simulink model "SEWSYS_Duplicate"  (Simulink 6.0)
settings: Solver=FixedStepDiscrete  SolverMode=SingleTasking  StartTime=0  StopTime=Q  FixedStep=1  RelTol=1e-3
PreLoadFcn:
  | helpdlg('After the simulation: run the file loadresults.m to load output data into MATLABs workspace. NOTE! All previous simulation data in subfolder Results is overwritten!')
values from neighbouring files (symbols this model uses):
  andpt = 1/3    (= 0.333333333333)    [constants.m]    (also in roadwear.m)
  andt = 0.15    [constants.m]    (also in roadwear.m = 0.1)
  baseflow = str2num(get(HH, 'String'))    [cal_inputs.m]
  BDT = [ ... (first row only)    [pollutants.m]
  BODofVS = 0.4    [sewageplant.m]
  delayinit = [zeros(1,nr_ex_H2O)]    [constants.m]
  Drainage = [ ... (first row only)    [pollutants.m]
  Faeces = [ ... (first row only)    [pollutants.m]
  fast = 0.7    [constants.m]    (also in roadwear.m = 0.5)
  Industry = [ ... (first row only)    [pollutants.m]
  K = a.*R.^b    [buildupwashoff.m]
  nr_ex_H2O = totnr-1    (= 20)    [cal_Prep.m]
  numberOfPersons = in_numberOfPersons    [cal_Prep.m]
  othermax = drydepmax*othera    [constants.m]
  ProcSS_bio = 0.01    [sewageplant.m]
  ProcSS_chem = 0.007    [sewageplant.m]
  ProcSS_presed = 0.025    [sewageplant.m]
  ProcSS_sand = 0.42*0.70    (= 0.294)    [sewageplant.m]
  ProcSS_screen = 0.185*0.85    (= 0.15725)    [sewageplant.m]
  roadaccmax = dryper*24*sph*fast*(p_tyrewear+p_roadwear+p_exhaust+p_breakwear+p_drydep+p_corrZn+p_oildischarge+p_catalyst)    [constants.m]
  roadkm = 63e9    (= 63000000000)    [constants.m]    (also in roadwear.m = 67000000000)
  roadrunpart = 1    [constants.m]
  roadwear = 130000    [constants.m]
  roofmax = (Znroofmax*RoofZna+Curoofmax*RoofCua)*roofrunpart+drydepmax*roofa    [constants.m]
  roofrunpart = 0.5    [constants.m]
  sec_per_ts = in_sec_per_ts    [cal_Prep.m]    (also in make_monthly_93_03.m = 600)
  spBiooxidBod = 0.5    [sewageplant.m]
  spBiored = 0.95    [sewageplant.m]
  spCcontent = 0.5424    [sewageplant.m]
  spChemFe = 0.171    [sewageplant.m]
  spChemicalPart = [ ... (first row only)    [sewageplant.m]
  spCODBOD = 2.51    [sewageplant.m]
  spDenSS = 0.25    [sewageplant.m]
  sph = 3600/sec_per_ts    [cal_Prep.m]
  spHeavym = [0.41 0.525 0.5 ... (first row only)    [sewageplant.m]
  spHjust = 1    [sewageplant.m]
  spN2ONpurEmitted = 0.0003    [sewageplant.m]
  spNemitted = 0.5    [sewageplant.m]
  spNitrif = 1.07    [sewageplant.m]
  spNpur = 1    [sewageplant.m]
  spOcontent = 0.3575    [sewageplant.m]
  spPBound = 0.97*0.5    (= 0.485)    [sewageplant.m]
  spPout = 0.38    [sewageplant.m]
  spPout1 = 0    [sewageplant.m]
  spVSofSS = 0.7    [sewageplant.m]
  SSred_bio = 0.65    [sewageplant.m]
  SSred_chem = 0.4    [sewageplant.m]
  SSred_presed = 0.75    [sewageplant.m]
  SSred_sand = 0.0032    [sewageplant.m]
  SSred_screen = 0.017    [sewageplant.m]
  SStoWater = 1E6    (= 1000000)    [sewageplant.m]
  totnr = 21    [cal_Prep.m]
  tyrewear = 9000    [constants.m]
  Urine = [ ... (first row only)    [pollutants.m]
  VSofSS_sand = 0.26    [sewageplant.m]
  VSofSS_screen = 0.60    (= 0.6)    [sewageplant.m]
  yearly_rain = in_yearly_rain    [cal_Prep.m]    (also in raininfo.m)
undefined symbols (not defined in the file or in its folder): brakep, catalystp, Curoofp, DiscIntNeverNeededParam, drydep, exhp, fkmday, init_init, init_time, nhv, oilp, othera, redu, roada, roadp, roadZna, roofa, RoofCua, RoofZna, sani, stormw, tota, tyrep, wetdep, Znroofp
libraries: simulink x2, SEWSYS_library x2
(part 2 of 2)

== system SEWSYS_Duplicate/Sewage plant/Sandpit/Separation/3-6 ==
  in_1 : Inport  Orientation=down  Port=1  LatchInput=off
  "in_2 " : Inport  Orientation=down  Port=2  LatchInput=off
  Ground2 : Ground  Orientation=down
  Mux : Mux  Orientation=down
  N-tot : MATLABFcn  Orientation=down  MATLABFcn=(u(1)-u(2)-u(3))*SSred_sand  OutputDimensions=1
  NH4 : Product  Orientation=down  SaturateOnIntegerOverflow=on  InputSameDT=on
  "NH4 " : Fcn  Orientation=down  Expr=u(2)
  NH5 : Product  Orientation=down  SaturateOnIntegerOverflow=on  InputSameDT=on
  NO3 : Fcn  Orientation=down  Expr=u(3)
  Sum : Sum  Orientation=down  Inputs=+++  SaturateOnIntegerOverflow=on  InputSameDT=on
  out_1 : Outport  Orientation=down  InitialOutput=0
  wires:
  Ground2/1 -> Mux/4
  NH5/1 -> Mux/3, Sum/3
  "in_2 "/1 -> N-tot/1, "NH4 "/1, NO3/1
  NO3/1 -> NH5/2
  "NH4 "/1 -> NH4/2
  Sum/1 -> Mux/1
  N-tot/1 -> Sum/1
  Mux/1 -> out_1/1
  in_1/1 -> NH4/1, NH5/1
  NH4/1 -> Sum/2, Mux/2

== system SEWSYS_Duplicate/Sewage plant/Sandpit/Separation/if u>0 then 1/u else 0 ==
  note: if u<=0, 0, else 1/u, end
  in_1 : Inport  Orientation=left  Port=1  LatchInput=off
  Constant : Constant  Orientation=left  Value=0
  Constant1 : Constant  Orientation=left
  Switch : Switch  Orientation=left  SaturateOnIntegerOverflow=on  InputSameDT=on
  Switch1 : Switch  Orientation=left  SaturateOnIntegerOverflow=on  InputSameDT=on
  inv. : Fcn  Orientation=left  Expr=1/u
  neg : Gain  Orientation=left  Gain=-1  SaturateOnIntegerOverflow=on
  neg1 : Gain  Orientation=left  Gain=-1  SaturateOnIntegerOverflow=on
  out_1 : Outport  Orientation=left  InitialOutput=0
  wires:
  Switch/1 -> out_1/1
  neg/1 -> Switch/2
  Constant/1 -> Switch/1
  inv./1 -> Switch/3
  Switch1/1 -> inv./1
  neg1/1 -> Switch1/2
  Constant1/1 -> Switch1/1
  in_1/1 -> neg/1, neg1/1, Switch1/3

== system SEWSYS_Duplicate/Sewage plant/Screen/Separation/3-6 ==
  in_1 : Inport  Orientation=down  Port=1  LatchInput=off
  "in_2 " : Inport  Orientation=down  Port=2  LatchInput=off
  Ground : Ground  Orientation=down
  Mux : Mux  Orientation=down
  N-tot : MATLABFcn  Orientation=down  MATLABFcn=(u(1)-u(2)-u(3))*SSred_screen  OutputDimensions=1
  NH4 : Product  Orientation=down  SaturateOnIntegerOverflow=on  InputSameDT=on
  "NH4 " : Fcn  Orientation=down  Expr=u(2)
  NH5 : Product  Orientation=down  SaturateOnIntegerOverflow=on  InputSameDT=on
  NO3 : Fcn  Orientation=down  Expr=u(3)
  Sum : Sum  Orientation=down  Inputs=+++  SaturateOnIntegerOverflow=on  InputSameDT=on
  out_1 : Outport  Orientation=down  InitialOutput=0
  wires:
  NH4/1 -> Mux/2, Sum/2
  in_1/1 -> NH5/1, NH4/1
  Mux/1 -> out_1/1
  N-tot/1 -> Sum/1
  Sum/1 -> Mux/1
  "NH4 "/1 -> NH4/2
  NO3/1 -> NH5/2
  "in_2 "/1 -> NO3/1, "NH4 "/1, N-tot/1
  NH5/1 -> Sum/3, Mux/3
  Ground/1 -> Mux/4

== system SEWSYS_Duplicate/Sewage plant/Screen/Separation/if u>0 then 1/u else 0 ==
  note: if u<=0, 0, else 1/u, end
  in_1 : Inport  Orientation=left  Port=1  LatchInput=off
  Constant : Constant  Orientation=left  Value=0
  Constant1 : Constant  Orientation=left
  Switch : Switch  Orientation=left  SaturateOnIntegerOverflow=on  InputSameDT=on
  Switch1 : Switch  Orientation=left  SaturateOnIntegerOverflow=on  InputSameDT=on
  inv. : Fcn  Orientation=left  Expr=1/u
  neg : Gain  Orientation=left  Gain=-1  SaturateOnIntegerOverflow=on
  neg1 : Gain  Orientation=left  Gain=-1  SaturateOnIntegerOverflow=on
  out_1 : Outport  Orientation=left  InitialOutput=0
  wires:
  Constant/1 -> Switch/1
  neg/1 -> Switch/2
  Switch/1 -> out_1/1
  inv./1 -> Switch/3
  Switch1/1 -> inv./1
  neg1/1 -> Switch1/2
  Constant1/1 -> Switch1/1
  in_1/1 -> neg/1, neg1/1, Switch1/3

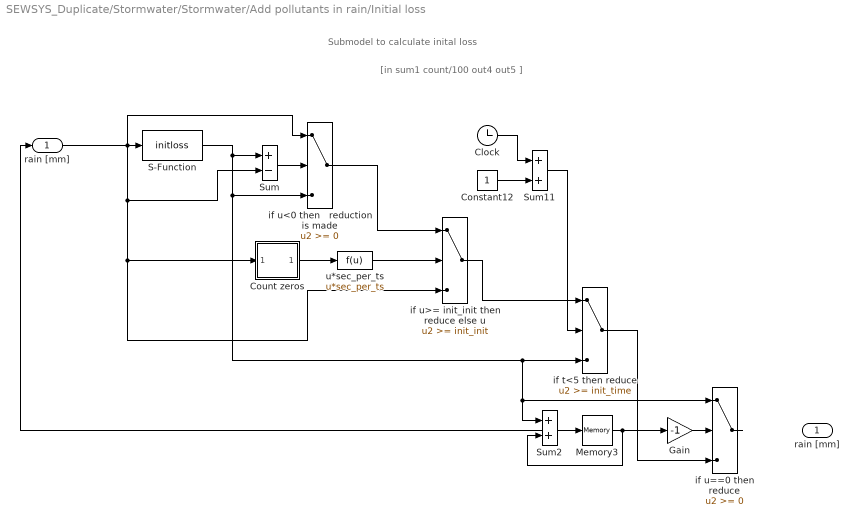
== system SEWSYS_Duplicate/Stormwater/Stormwater/Add pollutants in rain/Initial loss ==
  note: Submodel to calculate inital loss
  note: [in sum1 count/100 out4 out5 ]
  rain [mm] : Inport  Port=1  LatchInput=off
  Clock : Clock
      settings: Decimation=10
  Constant12 : Constant
  Count zeros : Subsystem
  Gain : Gain  Gain=-1  SaturateOnIntegerOverflow=on
  Memory3 : Memory
  S-Function : S-Function  FunctionName=initloss  Parameters=init
  Sum : Sum  Inputs=+-  SaturateOnIntegerOverflow=on  InputSameDT=on
  Sum11 : Sum  SaturateOnIntegerOverflow=on  InputSameDT=on
  Sum2 : Sum  SaturateOnIntegerOverflow=on  InputSameDT=on
  if t<5 then reduce : Switch  Threshold=init_time  SaturateOnIntegerOverflow=on  InputSameDT=on
  if u<0 then   reduction is made : Switch  SaturateOnIntegerOverflow=on  InputSameDT=on
  if u==0 then reduce : Switch  SaturateOnIntegerOverflow=on  InputSameDT=on
  if u>= init_init then reduce else u : Switch  Threshold=init_init  SaturateOnIntegerOverflow=on  InputSameDT=on
  u*sec_per_ts : Fcn  Expr=u*sec_per_ts
  rain [mm] : Outport
  wires:
  S-Function/1 -> Sum/1, if u<0 then   reduction is made/3, if t<5 then reduce/3, if u==0 then reduce/1, Sum2/1
  Sum11/1 -> if t<5 then reduce/2
  Sum/1 -> if u<0 then   reduction is made/2
  if u<0 then   reduction is made/1 -> if u>= init_init then reduce else u/1
  rain [mm]/1 -> Count zeros/1(In1), if u>= init_init then reduce else u/3, Sum/2, S-Function/1, if u<0 then   reduction is made/1
  Count zeros/1(Out1) -> u*sec_per_ts/1
  u*sec_per_ts/1 -> if u>= init_init then reduce else u/2
  Clock/1 -> Sum11/1
  Constant12/1 -> Sum11/2
  Gain/1 -> if u==0 then reduce/2
  if u==0 then reduce/1 -> rain [mm]/1
  Memory3/1 -> Gain/1, Sum2/2
  Sum2/1 -> Memory3/1
  if u>= init_init then reduce else u/1 -> if t<5 then reduce/1
  if t<5 then reduce/1 -> if u==0 then reduce/3

== system SEWSYS_Duplicate/Stormwater/Stormwater/Add pollutants in rain/wet deposition ==
  rain [mm] : Inport  Port=1  LatchInput=off
  Mux : Mux  Inputs=2
  Product1 : Product  SaturateOnIntegerOverflow=on  InputSameDT=on
  Product2 : Product  Inputs=*/  SaturateOnIntegerOverflow=on  InputSameDT=on
  To File : ToFile  Filename=Results\s_wetdep.mat  MatrixName=s_wetdep
      settings: Decimation=store1_yes
  To Workspace6 : ToWorkspace  VariableName=s_wetdep  SampleTime=-1  SaveFormat=Array
      settings: MaxDataPoints=lim_off
  rain mm/yr : Constant  Value=yearly_rain
  wet deposition ug/m2*yr : Constant  Value=wetdep
  rain [mm] pollutants [ug/m2] : Outport
  wires:
  rain [mm]/1 -> Product1/1, Mux/1
  Product2/1 -> Product1/2
  wet deposition ug/m2*yr/1 -> Product2/1
  rain mm/yr/1 -> Product2/2
  Product1/1 -> Mux/2
  Mux/1 -> rain [mm] pollutants [ug/m2]/1, To Workspace6/1, To File/1

== system SEWSYS_Duplicate/Stormwater/Stormwater/Rain -> Stormwater/other surfaces ==
  rain[mm] pollutants [ug/m2] : Inport  Port=1  LatchInput=off
  Demux2 : Demux  Outputs=[1 -1]
  Mux2 : Mux  Inputs=2
  Product1 : Product  SaturateOnIntegerOverflow=on  InputSameDT=on
  Sum : Sum  Inputs=|++  SaturateOnIntegerOverflow=on  InputSameDT=on
  To File : ToFile  Filename=Results\s_other.mat  MatrixName=s_other
      settings: Decimation=store1_yes
  To Workspace7 : ToWorkspace  VariableName=s_other  SampleTime=-1  SaveFormat=Array
      settings: MaxDataPoints=lim_off
  ackumulation and wash-off : Subsystem
  area [m2] : Constant  Value=othera
  dry deposition : Subsystem
  rain on other surfaces : Subsystem
  ug - g : Gain  Gain=0.000001  SaturateOnIntegerOverflow=on
  rain[m3] pollutants [g] : Outport
  wires:
  rain[mm] pollutants [ug/m2]/1 -> Demux2/1
  Mux2/1 -> rain[m3] pollutants [g]/1
  area [m2]/1 -> Product1/2
  Demux2/2 -> Product1/1
  Demux2/1 -> ackumulation and wash-off/1(rain [mm]), rain on other surfaces/1(rain [mm])
  dry deposition/1(pollutants [ug]) -> ackumulation and wash-off/2(pollutant [ug])
  Product1/1 -> Sum/2
  rain on other surfaces/1(rain [m3]) -> Mux2/1
  Sum/1 -> ug - g/1
  ug - g/1 -> Mux2/2
  ackumulation and wash-off/1(pollutants [ug]) -> Sum/1, To Workspace7/1, To File/1

== system SEWSYS_Duplicate/Stormwater/Stormwater/Rain -> Stormwater/road surfaces ==
  rain [mm] pollutants [ug/m2] : Inport  Port=1  LatchInput=off
  Demux1 : Demux  Outputs=[1 -1]
  Mux3 : Mux  Inputs=2
  Sum1 : Sum  Inputs=|++  SaturateOnIntegerOverflow=on  InputSameDT=on
  To File : ToFile  Filename=Results\s_road.mat  MatrixName=s_road
      settings: Decimation=store1_yes
  To Workspace7 : ToWorkspace  VariableName=s_road  SampleTime=-1  SaveFormat=Array
      settings: MaxDataPoints=lim_off
  To Workspace8 : ToWorkspace  VariableName=roadpoll  SampleTime=-1  SaveFormat=Array
      settings: MaxDataPoints=lim_off
  accumulation and wash-off : Subsystem
  pollutants on roads : Subsystem
  rain on road : Subsystem
  ug - g : Gain  Gain=0.000001  SaturateOnIntegerOverflow=on
  rain[m3] pollutants [g] : Outport
  wires:
  rain on road/1(rain [m3]) -> Mux3/1
  accumulation and wash-off/1(rain [mm]1) -> rain on road/1(rain [mm])
  Demux1/2 -> rain on road/2(pollutants [ug/m2])
  Demux1/1 -> accumulation and wash-off/1(rain [mm])
  rain [mm] pollutants [ug/m2]/1 -> Demux1/1
  Mux3/1 -> rain[m3] pollutants [g]/1
  rain on road/2(pollutants [ug]) -> Sum1/1
  accumulation and wash-off/2(pollutants [ug]) -> Sum1/2, To Workspace7/1, To File/1
  Sum1/1 -> ug - g/1
  ug - g/1 -> Mux3/2
  pollutants on roads/1(pollutants[ ug]) -> accumulation and wash-off/2(pollutant [ug]), To Workspace8/1

== system SEWSYS_Duplicate/Stormwater/Stormwater/Rain -> Stormwater/roofs ==
  note: Accumulates pollutants over time. Washes out during rain.
  rain [mm]  pollutants[ug/m2] : Inport  Port=1  LatchInput=off
  Demux : Demux  Outputs=[1 -1]
  Mux : Mux  Inputs=2
  Pollutants on roofs : Subsystem
  Product : Product  SaturateOnIntegerOverflow=on  InputSameDT=on
  Sum : Sum  Inputs=|++  SaturateOnIntegerOverflow=on  InputSameDT=on
  To File : ToFile  Filename=Results\s_roof.mat  MatrixName=s_roof
      settings: Decimation=store1_yes
  To Workspace7 : ToWorkspace  VariableName=s_roof  SampleTime=-1  SaveFormat=Array
      settings: MaxDataPoints=lim_off
  ackumulation and wash-off : Subsystem
  area [m2] : Constant  Value=roofa
  rain on roof surfaces : Subsystem
  ug - g : Gain  Gain=0.000001  SaturateOnIntegerOverflow=on
  rain[m3] pollutants [g] : Outport
  wires:
  Mux/1 -> rain[m3] pollutants [g]/1
  area [m2]/1 -> Product/2
  Demux/2 -> Product/1
  rain on roof surfaces/1(rain [m3]) -> Mux/1
  rain [mm]  pollutants[ug/m2]/1 -> Demux/1
  Product/1 -> Sum/2
  Sum/1 -> ug - g/1
  ug - g/1 -> Mux/2
  Demux/1 -> rain on roof surfaces/1(rain [mm]), ackumulation and wash-off/1(rain [mm])
  ackumulation and wash-off/1(pollutants [ug]) -> Sum/1, To Workspace7/1, To File/1
  Pollutants on roofs/1(pollutants [ug]) -> ackumulation and wash-off/2(pollutant [ug])

== system SEWSYS_Duplicate/Stormwater/Stormwater/Runoff/Make per second ==
  In1 : Inport  Port=1  LatchInput=off
  Demux : Demux  Outputs=[1 -1]
  Mux1 : Mux  Inputs=2
  g - g/s : Gain  Gain=1/sec_per_ts  SaturateOnIntegerOverflow=on
  m3 - m3/s : Gain  Gain=1/sec_per_ts  SaturateOnIntegerOverflow=on
  Out1 : Outport
  wires:
  In1/1 -> Demux/1
  Mux1/1 -> Out1/1
  Demux/1 -> m3 - m3/s/1
  m3 - m3/s/1 -> Mux1/1
  Demux/2 -> g - g/s/1
  g - g/s/1 -> Mux1/2

== system SEWSYS_Duplicate/Stormwater/Stormwater/Runoff/Subsystem1 ==
  In1 : Inport  Port=1  LatchInput=off
  Gain : Gain  Gain=sec_per_ts  SaturateOnIntegerOverflow=on
  Qut : Fcn  Expr=tota*K*u^(5/3)
  Sum : Sum  SaturateOnIntegerOverflow=on  InputSameDT=on
  Sum1 : Sum  Inputs=+-  SaturateOnIntegerOverflow=on  InputSameDT=on
  Sum2 : Sum  SaturateOnIntegerOverflow=on  InputSameDT=on
  Unit Delay1 : UnitDelay  Orientation=left
  Unit Delay2 : UnitDelay
  if u>0 then u else 1 : Subsystem
      mask Display: disp('1/u')
  y : Fcn  Expr=u/tota
  yprim : Fcn  Expr=u*sec_per_ts/tota/3
  Out1 : Outport
  wires:
  Qut/1 -> Sum1/2, Out1/1
  Unit Delay1/1 -> Sum2/2
  Sum2/1 -> Unit Delay1/1, y/1
  Gain/1 -> Sum2/1
  Sum1/1 -> Gain/1
  y/1 -> if u>0 then u else 1/1(in_1)
  yprim/1 -> Sum/1
  Sum/1 -> Qut/1
  if u>0 then u else 1/1(out_1) -> Unit Delay2/1
  Unit Delay2/1 -> Sum/2
  In1/1 -> Sum1/1, yprim/1

== system SEWSYS_Duplicate/Sewage plant/Biological stage/Predenitri- fication/N-org to NH4 through oxid to CO2/if u>0 then 1/u else 0 ==
  note: if u<=0, 0, else 1/u, end
  in_1 : Inport  Orientation=left  Port=1  LatchInput=off
  Constant : Constant  Orientation=left  Value=0
  Constant1 : Constant  Orientation=left
  Switch : Switch  Orientation=left  SaturateOnIntegerOverflow=on  InputSameDT=on
  Switch1 : Switch  Orientation=left  SaturateOnIntegerOverflow=on  InputSameDT=on
  inv. : Fcn  Orientation=left  Expr=1/u
  neg : Gain  Orientation=left  Gain=-1  SaturateOnIntegerOverflow=on
  out_1 : Outport  Orientation=left  InitialOutput=0
  wires:
  Constant1/1 -> Switch1/1
  in_1/1 -> Switch1/3, neg/1
  neg/1 -> Switch1/2, Switch/2
  Switch1/1 -> inv./1
  Switch/1 -> out_1/1
  inv./1 -> Switch/3
  Constant/1 -> Switch/1

== system SEWSYS_Duplicate/Sewage plant/Biological stage/Predenitri- fication/NH3 emissions from  aeration to nitrification  and degration of BOD./if u>0 then 1/u else 0 ==
  note: if u<=0, 0, else 1/u, end
  in_1 : Inport  Orientation=left  Port=1  LatchInput=off
  Constant : Constant  Orientation=left  Value=0
  Constant1 : Constant  Orientation=left
  Switch : Switch  Orientation=left  SaturateOnIntegerOverflow=on  InputSameDT=on
  Switch1 : Switch  Orientation=left  SaturateOnIntegerOverflow=on  InputSameDT=on
  inv. : Fcn  Orientation=left  Expr=1/u
  neg : Gain  Orientation=left  Gain=-1  SaturateOnIntegerOverflow=on
  out_1 : Outport  Orientation=left  InitialOutput=0
  wires:
  Constant1/1 -> Switch1/1
  in_1/1 -> Switch1/3, neg/1
  neg/1 -> Switch1/2, Switch/2
  Switch1/1 -> inv./1
  Switch/1 -> out_1/1
  inv./1 -> Switch/3
  Constant/1 -> Switch/1

== system SEWSYS_Duplicate/Sewage plant/Biological stage/Predenitri- fication/NH3 emissions from  aeration to nitrification  and degration of BOD./if u>0 then 1/u else 1 ==
  note: if u<=0, 0, else 1/u, end
  in_1 : Inport  Orientation=left  Port=1  LatchInput=off
  Constant : Constant  Orientation=left  Value=0
  Constant1 : Constant  Orientation=left
  Switch : Switch  Orientation=left  SaturateOnIntegerOverflow=on  InputSameDT=on
  Switch1 : Switch  Orientation=left  SaturateOnIntegerOverflow=on  InputSameDT=on
  inv. : Fcn  Orientation=left  Expr=1/u
  neg : Gain  Orientation=left  Gain=-1  SaturateOnIntegerOverflow=on
  out_1 : Outport  Orientation=left  InitialOutput=0
  wires:
  Constant1/1 -> Switch1/1
  in_1/1 -> Switch1/3, neg/1
  neg/1 -> Switch1/2, Switch/2
  Switch1/1 -> inv./1
  Switch/1 -> out_1/1
  inv./1 -> Switch/3
  Constant/1 -> Switch/1

== system SEWSYS_Duplicate/Sewage plant/Biological stage/Predenitri- fication/Nitrification/ denitrification/N-org to NH4 ==
  In1 : Inport  Orientation=down  Port=1  LatchInput=off
  In2 : Inport  Orientation=down  Port=2  LatchInput=off
  C-tot : Fcn  Orientation=down  Expr=u(10)
  Ctot degr. : Fcn  Orientation=down  Expr=u(10)
  N-org : Fcn  Orientation=down  Expr=u(3)-u(4)-u(5)
  N-org degraded  to NH4 : Product  Orientation=down  SaturateOnIntegerOverflow=on  InputSameDT=on
  NH4 increased : MATLABFcn  Orientation=down  MATLABFcn=[zeros(3,1); u ; zeros(17,1)]  OutputDimensions=totnr
  Part of C-tot degraded : Product  Orientation=down  SaturateOnIntegerOverflow=on  InputSameDT=on
  if u>0 then 1/u else 0 : Subsystem  Orientation=down
      mask Display: disp('1/u')
  Out1 : Outport  Orientation=down  InitialOutput=0
  wires:
  Ctot degr./1 -> Part of C-tot degraded/1
  In1/1 -> Ctot degr./1
  C-tot/1 -> if u>0 then 1/u else 0/1(in_1)
  if u>0 then 1/u else 0/1(out_1) -> Part of C-tot degraded/2
  In2/1 -> C-tot/1, N-org/1
  N-org/1 -> N-org degraded  to NH4/2
  N-org degraded  to NH4/1 -> NH4 increased/1
  NH4 increased/1 -> Out1/1
  Part of C-tot degraded/1 -> N-org degraded  to NH4/1

== system SEWSYS_Duplicate/Stormwater/Stormwater/Add pollutants in rain/Initial loss/Count zeros ==
  In1 : Inport  Port=1  LatchInput=off
  Constant13 : Constant  Value=0
  Constant8 : Constant
  Counter1 : Subsystem  TreatAsAtomicUnit=on
  Gain1 : Gain  Gain=-1  SaturateOnIntegerOverflow=on
  Memory1 : Memory
  if u== 0 then 1 else 1 : Switch  SaturateOnIntegerOverflow=on  InputSameDT=on
  Out1 : Outport
  wires:
  if u== 0 then 1 else 1/1 -> Counter1/Enable
  Counter1/1(Out1) -> Memory1/1
  Constant8/1 -> if u== 0 then 1 else 1/1
  Gain1/1 -> if u== 0 then 1 else 1/2
  Constant13/1 -> if u== 0 then 1 else 1/3
  In1/1 -> Gain1/1
  Memory1/1 -> Out1/1

== system SEWSYS_Duplicate/Stormwater/Stormwater/Rain -> Stormwater/other surfaces/ackumulation and wash-off ==
  rain [mm] : Inport  Port=1  LatchInput=off
  pollutant [ug] : Inport  Port=2  LatchInput=off
  Demux1 : Demux  Outputs=[1 -1]
  Mux : Mux  Inputs=2
  Mux1 : Mux  Inputs=3
  Specify initial condition here : UnitDelay  Orientation=left  X0=othermax
  Terminator : Terminator
  Unit Delay : UnitDelay  Orientation=left  X0=delayinit
  ackumulation Fcn1 : MATLABFcn  MATLABFcn=ackumulation  OutputDimensions=nr_ex_H2O
  deltaP : Scope
      settings: YMin=0  YMax=2250
  washoff Fcn : MATLABFcn  MATLABFcn=washoff  OutputDimensions=totnr
  pollutants [ug] : Outport
  wires:
  washoff Fcn/1 -> Demux1/1
  Demux1/2 -> deltaP/1, Unit Delay/1, pollutants [ug]/1
  Mux/1 -> washoff Fcn/1
  Unit Delay/1 -> Mux1/2
  Specify initial condition here/1 -> Mux1/3
  ackumulation Fcn1/1 -> Mux/2, Specify initial condition here/1
  Demux1/1 -> Terminator/1
  rain [mm]/1 -> Mux/1
  Mux1/1 -> ackumulation Fcn1/1
  pollutant [ug]/1 -> Mux1/1

== system SEWSYS_Duplicate/Stormwater/Stormwater/Rain -> Stormwater/other surfaces/dry deposition ==
  Product : Product  Inputs=*/  SaturateOnIntegerOverflow=on  InputSameDT=on
  Product1 : Product  SaturateOnIntegerOverflow=on  InputSameDT=on
  area m2 : Constant  Orientation=up  Value=othera
  timesteps/yr : Constant  Value=365*24*sph
  torrdep ug/m2*yr : Constant  Value=drydep
  pollutants [ug] : Outport
  wires:
  area m2/1 -> Product1/2
  Product1/1 -> pollutants [ug]/1
  Product/1 -> Product1/1
  torrdep ug/m2*yr/1 -> Product/1
  timesteps/yr/1 -> Product/2

== system SEWSYS_Duplicate/Stormwater/Stormwater/Rain -> Stormwater/other surfaces/rain on other surfaces ==
  rain [mm] : Inport  Port=1  LatchInput=off
  Product1 : Product  SaturateOnIntegerOverflow=on  InputSameDT=on
  area [m2] : Constant  Value=othera
  mm->m : Gain  Gain=0.001  SaturateOnIntegerOverflow=on
  rain [m3] : Outport
  wires:
  mm->m/1 -> Product1/1
  rain [mm]/1 -> mm->m/1
  area [m2]/1 -> Product1/2
  Product1/1 -> rain [m3]/1

== system SEWSYS_Duplicate/Stormwater/Stormwater/Rain -> Stormwater/road surfaces/accumulation and wash-off ==
  rain [mm] : Inport  Port=1  LatchInput=off
  pollutant [ug] : Inport  Port=2  LatchInput=off
  Demux1 : Demux  Outputs=[1 -1]
  Mux : Mux  Inputs=2
  Mux1 : Mux  Inputs=3
  Specify initial condition here : UnitDelay  Orientation=left  X0=roadaccmax
  To Workspace7 : ToWorkspace  VariableName=acc  SampleTime=-1  SaveFormat=Array
      settings: MaxDataPoints=lim_off
  Unit Delay : UnitDelay  Orientation=left  X0=delayinit
  ackumulation Fcn1 : MATLABFcn  MATLABFcn=ackumulation  OutputDimensions=nr_ex_H2O
  washoff Fcn : MATLABFcn  MATLABFcn=washoff  OutputDimensions=totnr
  rain [mm]1 : Outport
  pollutants [ug] : Outport  Port=2
  wires:
  Demux1/1 -> rain [mm]1/1
  pollutant [ug]/1 -> Mux1/1
  ackumulation Fcn1/1 -> Specify initial condition here/1, Mux/2, To Workspace7/1
  Specify initial condition here/1 -> Mux1/3
  Mux1/1 -> ackumulation Fcn1/1
  Unit Delay/1 -> Mux1/2
  Mux/1 -> washoff Fcn/1
  washoff Fcn/1 -> Demux1/1
  rain [mm]/1 -> Mux/1
  Demux1/2 -> Unit Delay/1, pollutants [ug]/1

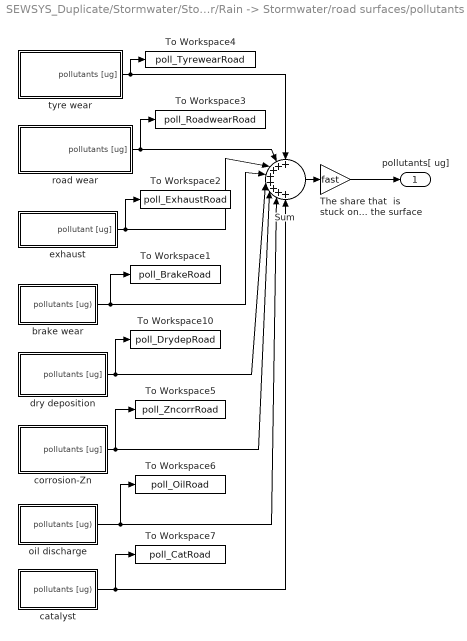
== system SEWSYS_Duplicate/Stormwater/Stormwater/Rain -> Stormwater/road surfaces/pollutants on roads ==
  Sum : Sum  Inputs=++++++++  SaturateOnIntegerOverflow=on  InputSameDT=on
  The share that  is stuck on the surface : Gain  Gain=fast  SaturateOnIntegerOverflow=on
  To Workspace1 : ToWorkspace  VariableName=poll_BrakeRoad  SampleTime=-1  SaveFormat=Array
      settings: MaxDataPoints=10
  To Workspace10 : ToWorkspace  VariableName=poll_DrydepRoad  SampleTime=-1  SaveFormat=Array
      settings: MaxDataPoints=10
  To Workspace2 : ToWorkspace  VariableName=poll_ExhaustRoad  SampleTime=-1  SaveFormat=Array
      settings: MaxDataPoints=10
  To Workspace3 : ToWorkspace  VariableName=poll_RoadwearRoad  SampleTime=-1  SaveFormat=Array
      settings: MaxDataPoints=10
  To Workspace4 : ToWorkspace  VariableName=poll_TyrewearRoad  SampleTime=-1  SaveFormat=Array
      settings: MaxDataPoints=10
  To Workspace5 : ToWorkspace  VariableName=poll_ZncorrRoad  SampleTime=-1  SaveFormat=Array
      settings: MaxDataPoints=10
  To Workspace6 : ToWorkspace  VariableName=poll_OilRoad  SampleTime=-1  SaveFormat=Array
      settings: MaxDataPoints=10
  To Workspace7 : ToWorkspace  VariableName=poll_CatRoad  SampleTime=-1  SaveFormat=Array
      settings: MaxDataPoints=10
  brake wear : Subsystem
  catalyst : Subsystem
  corrosion-Zn : Subsystem
  dry deposition : Subsystem
  exhaust : Subsystem
  oil discharge : Subsystem
  road wear : Subsystem
  tyre wear : Subsystem
  pollutants[ ug] : Outport
  wires:
  Sum/1 -> The share that  is stuck on the surface/1
  The share that  is stuck on the surface/1 -> pollutants[ ug]/1
  tyre wear/1(pollutants [ug]) -> Sum/1, To Workspace4/1
  road wear/1(pollutants [ug]) -> Sum/2, To Workspace3/1
  exhaust/1(pollutant [ug]) -> Sum/3, To Workspace2/1
  brake wear/1("pollutants [ug) ") -> Sum/4, To Workspace1/1
  dry deposition/1(pollutants [ug]) -> Sum/5, To Workspace10/1
  corrosion-Zn/1(pollutants [ug]) -> Sum/6, To Workspace5/1
  oil discharge/1("pollutants [ug) ") -> Sum/7, To Workspace6/1
  catalyst/1("pollutants [ug) ") -> Sum/8, To Workspace7/1

== system SEWSYS_Duplicate/Stormwater/Stormwater/Rain -> Stormwater/road surfaces/rain on road ==
  note: [m]
  rain [mm] : Inport  Port=1  LatchInput=off
  pollutants [ug/m2] : Inport  Port=2  LatchInput=off
  Gain : Gain  Gain=0.001  SaturateOnIntegerOverflow=on
  Product : Product  SaturateOnIntegerOverflow=on  InputSameDT=on
  Product1 : Product  SaturateOnIntegerOverflow=on  InputSameDT=on
  area [m2] : Constant  Value=roada
  rain [m3] : Outport
  pollutants [ug] : Outport  Port=2
  wires:
  Product1/1 -> pollutants [ug]/1
  pollutants [ug/m2]/1 -> Product1/2
  area [m2]/1 -> Product1/1, Product/2
  rain [mm]/1 -> Gain/1
  Gain/1 -> Product/1
  Product/1 -> rain [m3]/1

== system SEWSYS_Duplicate/Stormwater/Stormwater/Rain -> Stormwater/roofs/Pollutants on roofs ==
  Corrosion-Cu : Subsystem
  Corrosion-Zn : Subsystem
  Sum : Sum  Inputs=+++  SaturateOnIntegerOverflow=on  InputSameDT=on
  To Workspace10 : ToWorkspace  VariableName=poll_DrydepRoof  SampleTime=-1  SaveFormat=Array
      settings: MaxDataPoints=10
  To Workspace11 : ToWorkspace  VariableName=poll_ZnRoof  SampleTime=-1  SaveFormat=Array
      settings: MaxDataPoints=10
  To Workspace9 : ToWorkspace  VariableName=poll_CuRoof  SampleTime=-1  SaveFormat=Array
      settings: MaxDataPoints=10
  dry deposition : Subsystem
  pollutants [ug] : Outport
  wires:
  Sum/1 -> pollutants [ug]/1
  Corrosion-Cu/1(pollutants [ug]) -> Sum/2, To Workspace9/1
  Corrosion-Zn/1(pollutants [ug]) -> Sum/3, To Workspace11/1
  dry deposition/1(pollutants [ug]) -> Sum/1, To Workspace10/1

== system SEWSYS_Duplicate/Stormwater/Stormwater/Rain -> Stormwater/roofs/ackumulation and wash-off ==
  rain [mm] : Inport  Port=1  LatchInput=off
  pollutant [ug] : Inport  Port=2  LatchInput=off
  Demux1 : Demux  Outputs=[1 -1]
  Mux : Mux  Inputs=2
  Mux1 : Mux  Inputs=3
  Specify initial condition here : UnitDelay  Orientation=left  X0=roofmax
  Terminator : Terminator
  Unit Delay : UnitDelay  Orientation=left  X0=delayinit
  ackumulation Fcn1 : MATLABFcn  MATLABFcn=ackumulation  OutputDimensions=nr_ex_H2O
  deltaP : Scope
      settings: TimeRange=50  YMin=0  YMax=1e+07
  washoff Fcn : MATLABFcn  MATLABFcn=washoff  OutputDimensions=totnr
  pollutants [ug] : Outport
  wires:
  Demux1/1 -> Terminator/1
  ackumulation Fcn1/1 -> Mux/2, Specify initial condition here/1
  Specify initial condition here/1 -> Mux1/3
  Unit Delay/1 -> Mux1/2
  Mux/1 -> washoff Fcn/1
  Demux1/2 -> pollutants [ug]/1, Unit Delay/1, deltaP/1
  washoff Fcn/1 -> Demux1/1
  Mux1/1 -> ackumulation Fcn1/1
  pollutant [ug]/1 -> Mux1/1
  rain [mm]/1 -> Mux/1

== system SEWSYS_Duplicate/Stormwater/Stormwater/Rain -> Stormwater/roofs/rain on roof surfaces ==
  rain [mm] : Inport  Port=1  LatchInput=off
  Product1 : Product  SaturateOnIntegerOverflow=on  InputSameDT=on
  area [m2] : Constant  Value=roofa
  mm->m : Gain  Gain=0.001  SaturateOnIntegerOverflow=on
  rain [m3] : Outport
  wires:
  Product1/1 -> rain [m3]/1
  area [m2]/1 -> Product1/2
  rain [mm]/1 -> mm->m/1
  mm->m/1 -> Product1/1

== system SEWSYS_Duplicate/Stormwater/Stormwater/Runoff/Subsystem1/if u>0 then u else 1 ==
  note: if u<=0, 0, else u, end
  in_1 : Inport  Port=1  LatchInput=off
  Constant : Constant  Value=0
  Switch : Switch  SaturateOnIntegerOverflow=on  InputSameDT=on
  inv. : Fcn  Expr=u
  neg : Gain  Gain=-1  SaturateOnIntegerOverflow=on
  out_1 : Outport  InitialOutput=0
  wires:
  Switch/1 -> out_1/1
  Constant/1 -> Switch/1
  neg/1 -> Switch/2
  inv./1 -> Switch/3
  in_1/1 -> neg/1, inv./1

== system SEWSYS_Duplicate/Sewage plant/Biological stage/Predenitri- fication/Nitrification/ denitrification/N-org to NH4/if u>0 then 1/u else 0 ==
  note: if u<=0, 0, else 1/u, end
  in_1 : Inport  Orientation=left  Port=1  LatchInput=off
  Constant : Constant  Orientation=left  Value=0
  Constant1 : Constant  Orientation=left
  Switch : Switch  Orientation=left  SaturateOnIntegerOverflow=on  InputSameDT=on
  Switch1 : Switch  Orientation=left  SaturateOnIntegerOverflow=on  InputSameDT=on
  inv. : Fcn  Orientation=left  Expr=1/u
  neg : Gain  Orientation=left  Gain=-1  SaturateOnIntegerOverflow=on
  out_1 : Outport  Orientation=left  InitialOutput=0
  wires:
  Constant1/1 -> Switch1/1
  in_1/1 -> Switch1/3, neg/1
  neg/1 -> Switch1/2, Switch/2
  Switch1/1 -> inv./1
  Switch/1 -> out_1/1
  inv./1 -> Switch/3
  Constant/1 -> Switch/1

== system SEWSYS_Duplicate/Stormwater/Stormwater/Add pollutants in rain/Initial loss/Count zeros/Counter1 ==
  Enable : EnablePort  StatesWhenEnabling=reset
  Constant7 : Constant
  Discrete-Time Integrator : DiscreteIntegrator  InitialCondition=1  ICPrevOutput=DiscIntNeverNeededParam  ICPrevScaledInput=DiscIntNeverNeededParam
  Out1 : Outport  InitialOutput=0
  wires:
  Discrete-Time Integrator/1 -> Out1/1
  Constant7/1 -> Discrete-Time Integrator/1

== system SEWSYS_Duplicate/Stormwater/Stormwater/Rain -> Stormwater/road surfaces/pollutants on roads/brake wear ==
  note: [ug/fkm]
  Product : Product  Inputs=*/  SaturateOnIntegerOverflow=on  InputSameDT=on
  Product1 : Product  SaturateOnIntegerOverflow=on  InputSameDT=on
  fordonskm/day : Constant  Value=fkmday
  pollutants from brakes : Constant  Value=brakep
  timesteps/day : Constant  Value=24*sph
  "pollutants [ug) " : Outport
  wires:
  Product1/1 -> "pollutants [ug) "/1
  pollutants from brakes/1 -> Product1/2
  fordonskm/day/1 -> Product/1
  timesteps/day/1 -> Product/2
  Product/1 -> Product1/1

== system SEWSYS_Duplicate/Stormwater/Stormwater/Rain -> Stormwater/road surfaces/pollutants on roads/catalyst ==
  note: [ug/fkm]
  Product : Product  Inputs=*/  SaturateOnIntegerOverflow=on  InputSameDT=on
  Product1 : Product  SaturateOnIntegerOverflow=on  InputSameDT=on
  fordonskm/day : Constant  Value=fkmday
  pollutants from catalysts : Constant  Value=catalystp
  timesteps/day : Constant  Value=24*sph
  "pollutants [ug) " : Outport
  wires:
  Product1/1 -> "pollutants [ug) "/1
  pollutants from catalysts/1 -> Product1/2
  fordonskm/day/1 -> Product/1
  timesteps/day/1 -> Product/2
  Product/1 -> Product1/1

== system SEWSYS_Duplicate/Stormwater/Stormwater/Rain -> Stormwater/road surfaces/pollutants on roads/corrosion-Zn ==
  Product : Product  SaturateOnIntegerOverflow=on  InputSameDT=on
  area [m2] : Constant  Value=roadZna
  avrunnen andel : Gain  Gain=roadrunpart  SaturateOnIntegerOverflow=on
  pollutants from  zink surface : Subsystem
  pollutants [ug] : Outport
  wires:
  Product/1 -> pollutants [ug]/1
  pollutants from  zink surface/1("[ug/m2]") -> avrunnen andel/1
  avrunnen andel/1 -> Product/1
  area [m2]/1 -> Product/2

== system SEWSYS_Duplicate/Stormwater/Stormwater/Rain -> Stormwater/road surfaces/pollutants on roads/dry deposition ==
  Product : Product  Inputs=*/  SaturateOnIntegerOverflow=on  InputSameDT=on
  Product1 : Product  SaturateOnIntegerOverflow=on  InputSameDT=on
  area m2 : Constant  Orientation=up  Value=roada
  timesteps/yr : Constant  Value=365*24*sph
  torrdep ug/m2*yr : Constant  Value=drydep
  pollutants [ug] : Outport
  wires:
  timesteps/yr/1 -> Product/2
  torrdep ug/m2*yr/1 -> Product/1
  Product/1 -> Product1/1
  Product1/1 -> pollutants [ug]/1
  area m2/1 -> Product1/2

== system SEWSYS_Duplicate/Stormwater/Stormwater/Rain -> Stormwater/road surfaces/pollutants on roads/exhaust ==
  Product : Product  SaturateOnIntegerOverflow=on  InputSameDT=on
  Product1 : Product  Inputs=*/  SaturateOnIntegerOverflow=on  InputSameDT=on
  fordonskm/day : Constant  Value=fkmday
  pollutant [ug/fkm] : Constant  Value=exhp
  timesteps/day : Constant  Value=24*sph
  pollutant [ug] : Outport
  wires:
  fordonskm/day/1 -> Product1/1
  timesteps/day/1 -> Product1/2
  Product/1 -> pollutant [ug]/1
  pollutant [ug/fkm]/1 -> Product/2
  Product1/1 -> Product/1

== system SEWSYS_Duplicate/Stormwater/Stormwater/Rain -> Stormwater/road surfaces/pollutants on roads/oil discharge ==
  note: [ug/fkm]
  Product : Product  Inputs=*/  SaturateOnIntegerOverflow=on  InputSameDT=on
  Product1 : Product  SaturateOnIntegerOverflow=on  InputSameDT=on
  fordonskm/day : Constant  Value=fkmday
  pollutants from oil : Constant  Value=oilp
  timesteps/day : Constant  Value=24*sph
  "pollutants [ug) " : Outport
  wires:
  Product/1 -> Product1/1
  timesteps/day/1 -> Product/2
  fordonskm/day/1 -> Product/1
  pollutants from oil/1 -> Product1/2
  Product1/1 -> "pollutants [ug) "/1

== system SEWSYS_Duplicate/Stormwater/Stormwater/Rain -> Stormwater/road surfaces/pollutants on roads/road wear ==
  note: kilos of road material
      | per time unit
  Fcn : Fcn  Expr=1-u[1]
  Product : Product  Inputs=3  SaturateOnIntegerOverflow=on  InputSameDT=on
  Product1 : Product  Inputs=3  SaturateOnIntegerOverflow=on  InputSameDT=on
  Product2 : Product  SaturateOnIntegerOverflow=on  InputSameDT=on
  Product3 : Product  Inputs=*/  SaturateOnIntegerOverflow=on  InputSameDT=on
  Road wear : Subsystem
  Sum : Sum  Inputs=|++  SaturateOnIntegerOverflow=on  InputSameDT=on
  andel tunga fordon : Constant  Value=nhv
  fordonskm/day : Constant  Value=fkmday
  mg->ug : Gain  Gain=1000  SaturateOnIntegerOverflow=on
  "pollutants in road mat. ppm " : Constant  Orientation=up  Value=roadp
  timesteps/day : Constant  Value=24*sph
  pollutants [ug] : Outport
  wires:
  mg->ug/1 -> pollutants [ug]/1
  Road wear/1(vägslitage kg/tfkm) -> Product/1
  Road wear/2(vägslitage kg/pbkm) -> Product1/3
  Sum/1 -> Product2/1
  Product/1 -> Sum/1
  Product1/1 -> Sum/2
  Fcn/1 -> Product1/2
  andel tunga fordon/1 -> Fcn/1, Product/2
  "pollutants in road mat. ppm "/1 -> Product2/2
  Product2/1 -> mg->ug/1
  timesteps/day/1 -> Product3/2
  fordonskm/day/1 -> Product3/1
  Product3/1 -> Product/3, Product1/1

== system SEWSYS_Duplicate/Stormwater/Stormwater/Rain -> Stormwater/road surfaces/pollutants on roads/tyre wear ==
  note: [mg]
  note: Kilos of tyre per
      | time unit
  Fcn : Fcn  Expr=1-u[1]
  Gain : Gain  Gain=1000  SaturateOnIntegerOverflow=on
  Product : Product  Inputs=3  SaturateOnIntegerOverflow=on  InputSameDT=on
  Product1 : Product  Inputs=3  SaturateOnIntegerOverflow=on  InputSameDT=on
  Product2 : Product  SaturateOnIntegerOverflow=on  InputSameDT=on
  Product3 : Product  Inputs=*/  SaturateOnIntegerOverflow=on  InputSameDT=on
  Sum : Sum  Inputs=|++  SaturateOnIntegerOverflow=on  InputSameDT=on
  andel tunga fordon : Constant  Value=nhv
  fordonskm/day : Constant  Value=fkmday
  pollutants in tyre  [ppm] : Constant  Orientation=up  Value=tyrep
  timesteps/day : Constant  Value=24*sph
  tyre wear : Subsystem
  pollutants [ug] : Outport
  wires:
  Gain/1 -> pollutants [ug]/1
  pollutants in tyre  [ppm]/1 -> Product2/2
  Sum/1 -> Product2/1
  andel tunga fordon/1 -> Product/2, Fcn/1
  Fcn/1 -> Product1/2
  Product1/1 -> Sum/2
  Product/1 -> Sum/1
  Product2/1 -> Gain/1
  tyre wear/1(tyre wear [kg/tfkm]) -> Product/1
  tyre wear/2(tyre wear [kg/pbkm]) -> Product1/3
  timesteps/day/1 -> Product3/2
  fordonskm/day/1 -> Product3/1
  Product3/1 -> Product/3, Product1/1

== system SEWSYS_Duplicate/Stormwater/Stormwater/Rain -> Stormwater/roofs/Pollutants on roofs/Corrosion-Cu ==
  Product : Product  SaturateOnIntegerOverflow=on  InputSameDT=on
  Product1 : Product  Inputs=*/  SaturateOnIntegerOverflow=on  InputSameDT=on
  area [m2] : Constant  Value=RoofCua
  avrunnen andel : Gain  Gain=roofrunpart  SaturateOnIntegerOverflow=on
  g/m2->ug/m2 : Gain  Gain=1000000  SaturateOnIntegerOverflow=on
  pollutants [g/m2*yr] : Constant  Value=Curoofp
  timesteps/yr : Constant  Value=365*24*sph
  pollutants [ug] : Outport
  wires:
  pollutants [g/m2*yr]/1 -> g/m2->ug/m2/1
  Product1/1 -> avrunnen andel/1
  g/m2->ug/m2/1 -> Product1/1
  timesteps/yr/1 -> Product1/2
  area [m2]/1 -> Product/2
  avrunnen andel/1 -> Product/1
  Product/1 -> pollutants [ug]/1

== system SEWSYS_Duplicate/Stormwater/Stormwater/Rain -> Stormwater/roofs/Pollutants on roofs/Corrosion-Zn ==
  Product : Product  SaturateOnIntegerOverflow=on  InputSameDT=on
  Product1 : Product  Inputs=*/  SaturateOnIntegerOverflow=on  InputSameDT=on
  area [m2] : Constant  Value=RoofZna
  avrunnen andel : Gain  Gain=roofrunpart  SaturateOnIntegerOverflow=on
  g/m2->ug/m2 : Gain  Gain=1000000  SaturateOnIntegerOverflow=on
  pollutants [g/m2*yr] : Constant  Value=Znroofp
  timesteps/yr : Constant  Value=365*24*sph
  pollutants [ug] : Outport
  wires:
  Product1/1 -> avrunnen andel/1
  timesteps/yr/1 -> Product1/2
  pollutants [g/m2*yr]/1 -> g/m2->ug/m2/1
  g/m2->ug/m2/1 -> Product1/1
  Product/1 -> pollutants [ug]/1
  avrunnen andel/1 -> Product/1
  area [m2]/1 -> Product/2

== system SEWSYS_Duplicate/Stormwater/Stormwater/Rain -> Stormwater/roofs/Pollutants on roofs/dry deposition ==
  Product : Product  Inputs=*/  SaturateOnIntegerOverflow=on  InputSameDT=on
  Product1 : Product  SaturateOnIntegerOverflow=on  InputSameDT=on
  area m2 : Constant  Orientation=up  Value=roofa
  timesteps/yr : Constant  Value=365*24*sph
  torrdep ug/m2*yr : Constant  Value=drydep
  pollutants [ug] : Outport
  wires:
  timesteps/yr/1 -> Product/2
  torrdep ug/m2*yr/1 -> Product/1
  Product/1 -> Product1/1
  Product1/1 -> pollutants [ug]/1
  area m2/1 -> Product1/2

== system SEWSYS_Duplicate/Stormwater/Stormwater/Rain -> Stormwater/road surfaces/pollutants on roads/corrosion-Zn/pollutants from  zink surface ==
  Product : Product  Inputs=*/  SaturateOnIntegerOverflow=on  InputSameDT=on
  g/m2->ug/m2 : Gain  Gain=1000000  SaturateOnIntegerOverflow=on
  pollutants [g/m2*yr] : Constant  Value=Znroofp
  timesteps/yr : Constant  Value=365*24*sph
  "[ug/m2]" : Outport
  wires:
  Product/1 -> "[ug/m2]"/1
  timesteps/yr/1 -> Product/2
  pollutants [g/m2*yr]/1 -> g/m2->ug/m2/1
  g/m2->ug/m2/1 -> Product/1

== system SEWSYS_Duplicate/Stormwater/Stormwater/Rain -> Stormwater/road surfaces/pollutants on roads/road wear/Road wear ==
  Constant : Constant  Value=[andt roadkm roadwear andpt]
  Fcn : Fcn  Expr=(u[3]*u[4])/(u[1]*u[2])
  Fcn1 : Fcn  Expr=(u[3]*(1-u[4]))/(u[2]*(1-u[1]))
  Gain : Gain  Gain=[1 1 1000 1]  SaturateOnIntegerOverflow=on
  vägslitage kg/tfkm : Outport
  vägslitage kg/pbkm : Outport  Port=2
  wires:
  Gain/1 -> Fcn1/1, Fcn/1
  Constant/1 -> Gain/1
  Fcn/1 -> vägslitage kg/tfkm/1
  Fcn1/1 -> vägslitage kg/pbkm/1

== system SEWSYS_Duplicate/Stormwater/Stormwater/Rain -> Stormwater/road surfaces/pollutants on roads/tyre wear/tyre wear ==
  note: change of units
      | tons-kg
  Constant : Constant  Value=[andt roadkm tyrewear andpt]
  Fcn : Fcn  Expr=(u[3]*u[4])/(u[1]*u[2])
  Fcn1 : Fcn  Expr=(u[3]*(1-u[4]))/(u[2]*(1-u[1]))
  Gain : Gain  Gain=[1 1 1000 1]  SaturateOnIntegerOverflow=on
  tyre wear [kg/tfkm] : Outport
  tyre wear [kg/pbkm] : Outport  Port=2
  wires:
  Gain/1 -> Fcn1/1, Fcn/1
  Constant/1 -> Gain/1
  Fcn/1 -> tyre wear [kg/tfkm]/1
  Fcn1/1 -> tyre wear [kg/pbkm]/1
